simulink model "Ex_4"  (R2020a)
settings: Solver=VariableStepAuto  StartTime=0.0  StopTime=5  RelTol=1e-3
values from neighbouring files (symbols this model uses):
  B = 0.008    [m4.m]    (also in m5.m = 0)
  J = 0.093    [m4.m]    (also in m5.m = 1)
  K = 0.55    [m4.m]
  La = 0.046    [m4.m]    (also in m5.m = 0.012)
  Load = 2.5    [m4.m]
  Ra = 1    [m4.m]    (also in m5.m = 0.6)
  Va = 220    [m4.m]    (also in m5.m = 240)
settings Model: Creator=abhin  LastModifiedBy=abhin

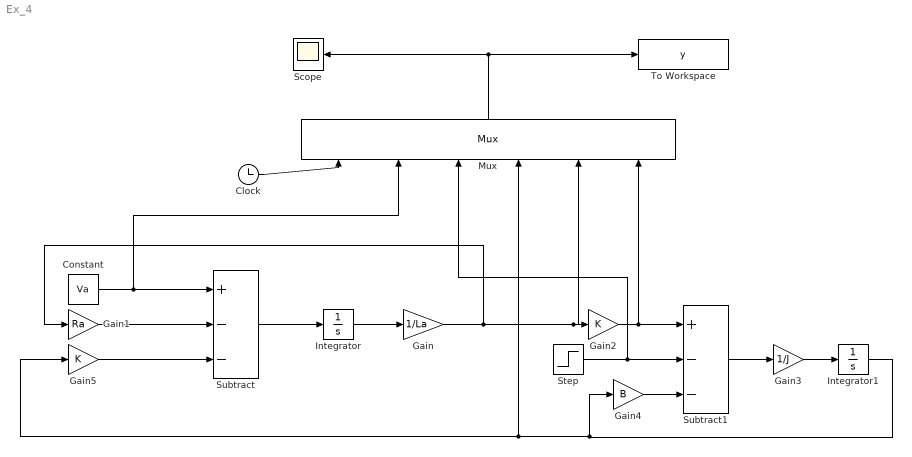
== system Ex_4 ==
  Clock : Clock
  Constant : Constant  Value=Va  SampleTime=1e-3
  Gain : Gain  Gain=1/La
  Gain1 : Gain  Gain=Ra
  Gain2 : Gain  Gain=K
  Gain3 : Gain  Gain=1/J
  Gain4 : Gain  Gain=B
  Gain5 : Gain  Gain=K
  Integrator : Integrator
  Integrator1 : Integrator
  Mux : Mux  Inputs=6
  Scope : Scope
  Step : Step  Time=2  After=8*Load  SampleTime=1e-3
  Subtract : Sum  Inputs=+--
  Subtract1 : Sum  Inputs=+--
  To Workspace : ToWorkspace  VariableName=y  SaveFormat=Structure  SampleTime=-1
      settings: Save2DSignal=2-D array (concatenate along first dimension)
  wires:
  Constant/1 -> Subtract/1, Mux/2
  Subtract/1 -> Integrator/1
  Integrator/1 -> Gain/1
  Gain1/1 -> Subtract/2
  Gain/1 -> Mux/5, Gain2/1, Gain1/1
  Gain5/1 -> Subtract/3
  Gain2/1 -> Subtract1/1, Mux/6
  Gain3/1 -> Integrator1/1
  Subtract1/1 -> Gain3/1
  Integrator1/1 -> Mux/4, Gain5/1, Gain4/1
  Gain4/1 -> Subtract1/3
  Clock/1 -> Mux/1
  Mux/1 -> Scope/1, To Workspace/1
  Step/1 -> Mux/3, Subtract1/2
